simulink model "mdaq_analog"  (R2013a)
settings: Solver=FixedStepDiscrete  StartTime=0.0  StopTime=10  RelTol=1e-3
libraries: microdaq_lib x2
settings Model: Creator=peselnikmg  LastModifiedBy=w530
settings DataIOCC: LimitDataPoints=off  SignalLoggingSaveFormat=ModelDataLogs  SaveOutput=off  SignalLogging=off  DSMLogging=off  SaveTime=off
settings OptimizationCC: InlineParams=on  OptimizeModelRefInitCode=on  LifeSpan=1
settings HardwareCC: ProdBitPerLong=40  ProdLargestAtomicInteger=Integer  ProdIntDivRoundTo=Zero  ProdEndianess=LittleEndian  ProdHWDeviceType=Texas Instruments->C6000
settings RTWCC: SystemTargetFile=microdaq.tlc  TemplateMakefile=microdaq.tmf  PostCodeGenCommand=microdaq_postcodegen(buildInfo)  Description=MicroDAQ Real-Time Measurement System  GenerateReport=on  ProcessScript=microdaq_make_rtw_hook  IncludeHyperlinkInReport=on
settings CodeAppCC: IgnoreCustomStorageClasses=off
settings STFCustomTargetCC: CodeReplacementLibrary=TI C674x  CombineOutputUpdateFcns=on  ERTCustomFileBanners=on  SupportContinuousTime=off  SupportNonInlinedSFcns=off  MATLABClassNameForMDSCustomization=Simulink.SoftwareTarget.ERTCustomization  SystemTargetFile=microdaq.tlc
settings ERTTargetCC: CodeReplacementLibrary=TI C674x  GenerateSampleERTMain=off  ParMdlRefBuildCompliant=off  CompOptLevelCompliant=off  ConcurrentExecutionCompliant=off  ERTFirstTimeCompliant=off  ModelStepFunctionPrototypeControlCompliant=off  CPPClassGenCompliant=off  ERTCustomFileTemplate=microdaq_main.tlc

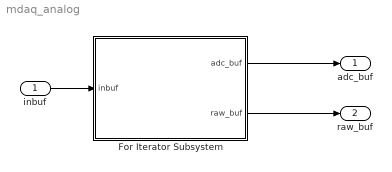
== system mdaq_analog ==
  inbuf : Inport  OutDataTypeStr=double
  For Iterator Subsystem : Subsystem  TreatAsAtomicUnit=on  mask{BufSize=100}
      mask prompts: BufSize "Buffer size:"
      mask Display: fprintf('Buffer size: %d\n',BufSize);
  adc_buf : Outport  SampleTime=0.1
  raw_buf : Outport  Port=2  SampleTime=0.1
  wires:
  For Iterator Subsystem/1(adc_buf) -> adc_buf/1
  For Iterator Subsystem/2(raw_buf) -> raw_buf/1
  inbuf/1 -> For Iterator Subsystem/1(inbuf)

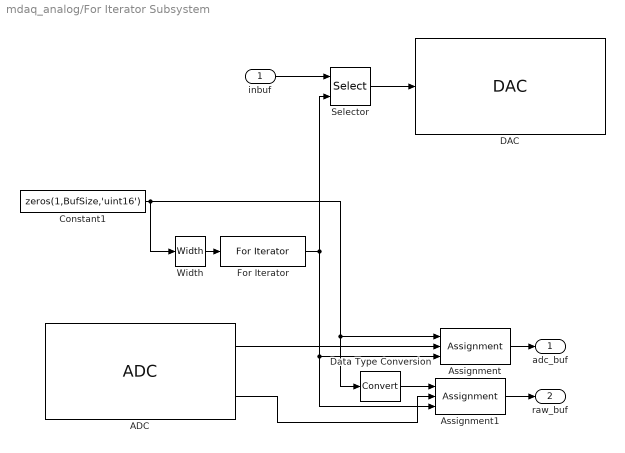
== system mdaq_analog/For Iterator Subsystem ==
  inbuf : Inport
  ADC : microdaq_lib/ADC  pConverter=ADC01 - 8 channel, 166ksps, 12-bit, -/+10V range  pChannel=1  pChannelCount=ones([1 1 ])  pRange=10V  pPolarity=Bipolar  pMode=Single-ended  SampleTime=-1
  Assignment : Assignment  IndexOptions=Index vector (port)  Indices=1  OutputSizes=100
  Assignment1 : Assignment  IndexOptions=Index vector (port)  Indices=1  OutputSizes=100
  Constant1 : Constant  Value=zeros(1,BufSize,'uint16')
  DAC : microdaq_lib/DAC  pConverter=DAC01 - 8 channel, 12-bit, 0-5V range  pChannel=1  pChannelCount=ones([1 1 ])  pMode=Sequential  pModeTrig=Software  pTermAll=on  pTerm=0  SampleTime=-1
  Data Type Conversion : DataTypeConversion
  For Iterator : ForIterator  IterationSource=external  IterationLimit=100
  Selector : Selector  InputPortWidth=BufSize  IndexOptions=Index vector (port)  Indices=[1 3]  OutputSizes=1
  Width : Width
  adc_buf : Outport
  raw_buf : Outport  Port=2
  wires:
  Assignment/1 -> adc_buf/1
  For Iterator/1 -> Selector/2, Assignment1/3, Assignment/3
  Constant1/1 -> Width/1, Data Type Conversion/1, Assignment/1
  Width/1 -> For Iterator/1
  Assignment1/1 -> raw_buf/1
  Data Type Conversion/1 -> Assignment1/1
  inbuf/1 -> Selector/1
  Selector/1 -> DAC/1
  ADC/2 -> Assignment1/2
  ADC/1 -> Assignment/2
